simulink model "DualEMDrive3EMRear"  (R2026b)
settings: Solver=VariableStepAuto
undefined symbols (not defined in the file): PlntEMWhlGearRatioRL, PlntEMWhlGearRatioRR
libraries: autolibsharedcoupling x2
settings Model: ModifiedByFormat=The MathWorks, Inc.  Creator=The MathWorks, Inc.  LastModifiedBy=The MathWorks, Inc.
settings OptimizationCC: ReuseModelBlockBuffer=off

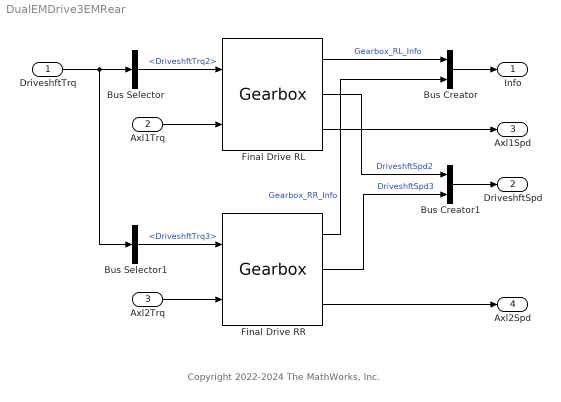
== system DualEMDrive3EMRear ==
  note: Copyright 2022-2024 The MathWorks, Inc.
  DriveshftTrq : Inport
  Axl1Trq : Inport  Port=2
  Axl2Trq : Inport  Port=3
  Bus Creator : BusCreator  Inputs=2
  Bus Creator1 : BusCreator  Inputs=2
  Bus Selector : BusSelector  OutputSignals=DriveshftTrq2
  Bus Selector1 : BusSelector  OutputSignals=DriveshftTrq3
  Final Drive RL : autolibsharedcoupling/Gearbox  port_config=Simulink  input_config=Torque input - velocity output  DiffEffModelPopup=Constant  InterpMethod=Flat  dirSwitch=on  extTamb=off  N=PlntEMWhlGearRatioRL  J1=PlntEMWhlGearInInertiaRL  J2=PlntEMWhlGearOutInertiaRL  b1=PlntEMWhlGearInDampRL  b2=PlntEMWhlGearOutDampRL  theta1_o=0  w1_o=PlntEMWhlGearInInitVelRL  eta=PlntEMWhlGearEffRL  eta_tbl=reshape([0.64 0.76 0.8 0.81 0.83 0.84 0.84 0.56 0.73 0.78 0.8 0.83 0.84 0.84 0.54 0.71 0.77 0.8 0.82 0.84 0.84 0.53 0.71 0.77 0.8 0.83 0.84 0.84 0.51 0.71 0.77 0.8 0.83 0.84 0.85 0.52 0.7 0.77 0.8 0.83 0.84 0.85 0.51 0.71 0.76 0.79 0.83 0.84 0.85 0.5 0.69 0.76 0.79 0.82 0.84 0.85 0.45 0.68 0.75 0.78 0.82 0.84 0.85 0.43 0.67 0.74 0.78 0.81 0.83 0.84 0.38 0.63 0.71 0.75 0.8 0.82 0.83 0.81 0.86 0.88 0.89 0.89 0.89 0.9 0.77 0.85 0.87 0.88 0.89 0.9 0.9 0.72 0.82 0.86 0.87 0.88 0.89 0.9 0.68 0.8 0.84 0.86 0.88 0.89 0.89 0.67 0.8 0.84 0.86 0.88 0.89 0.9 0.67 0.8 0.84 0.86 0.88 0.89 0.9 0.65 0.8 0.84 0.86 0.88 0.89 0.9 0.64 0.79 0.83 0.86 0.88 0.89 0.9 0.63 0.78 0.83 0.86 0.88 0.89 0.9 0.59 0.76 0.82 0.85 0.87 0.89 0.9 0.53 0.73 0.8 0.83 0.86 0.88 0.89], 7, 11, 2)  Trq_bpts=[25, 50, 75, 100, 150, 200, 250]  omega_bpts=[52.4 78.5 105 131 157 183 209 262 314 419 524]  Temp_bpts=[290 358]  Tamb=297.15  blkID=0  aMode=1
      settings: LibrarySourceBlock=autolibcoupling/Gearbox
  Final Drive RR : autolibsharedcoupling/Gearbox  port_config=Simulink  input_config=Torque input - velocity output  DiffEffModelPopup=Constant  InterpMethod=Flat  dirSwitch=on  extTamb=off  N=PlntEMWhlGearRatioRR  J1=PlntEMWhlGearInInertiaRR  J2=PlntEMWhlGearOutInertiaRR  b1=PlntEMWhlGearInDampRR  b2=PlntEMWhlGearOutDampRR  theta1_o=0  w1_o=PlntEMWhlGearInInitVelRR  eta=PlntEMWhlGearEffRR  eta_tbl=reshape([0.64 0.76 0.8 0.81 0.83 0.84 0.84 0.56 0.73 0.78 0.8 0.83 0.84 0.84 0.54 0.71 0.77 0.8 0.82 0.84 0.84 0.53 0.71 0.77 0.8 0.83 0.84 0.84 0.51 0.71 0.77 0.8 0.83 0.84 0.85 0.52 0.7 0.77 0.8 0.83 0.84 0.85 0.51 0.71 0.76 0.79 0.83 0.84 0.85 0.5 0.69 0.76 0.79 0.82 0.84 0.85 0.45 0.68 0.75 0.78 0.82 0.84 0.85 0.43 0.67 0.74 0.78 0.81 0.83 0.84 0.38 0.63 0.71 0.75 0.8 0.82 0.83 0.81 0.86 0.88 0.89 0.89 0.89 0.9 0.77 0.85 0.87 0.88 0.89 0.9 0.9 0.72 0.82 0.86 0.87 0.88 0.89 0.9 0.68 0.8 0.84 0.86 0.88 0.89 0.89 0.67 0.8 0.84 0.86 0.88 0.89 0.9 0.67 0.8 0.84 0.86 0.88 0.89 0.9 0.65 0.8 0.84 0.86 0.88 0.89 0.9 0.64 0.79 0.83 0.86 0.88 0.89 0.9 0.63 0.78 0.83 0.86 0.88 0.89 0.9 0.59 0.76 0.82 0.85 0.87 0.89 0.9 0.53 0.73 0.8 0.83 0.86 0.88 0.89], 7, 11, 2)  Trq_bpts=[25, 50, 75, 100, 150, 200, 250]  omega_bpts=[52.4 78.5 105 131 157 183 209 262 314 419 524]  Temp_bpts=[290 358]  Tamb=297.15  blkID=0  aMode=1
      settings: LibrarySourceBlock=autolibcoupling/Gearbox
  Info : Outport
  DriveshftSpd : Outport  Port=2
  Axl1Spd : Outport  Port=3
  Axl2Spd : Outport  Port=4
  wires:
  Bus Creator/1 -> Info/1
  Axl2Trq/1 -> Final Drive RR/2
  Final Drive RR/3 -> Axl2Spd/1
  Axl1Trq/1 -> Final Drive RL/2
  Final Drive RL/3 -> Axl1Spd/1
  Bus Selector1/1 -> Final Drive RR/1  "<DriveshftTrq3>"
  Final Drive RR/2 -> Bus Creator1/2  "DriveshftSpd3"
  Bus Creator1/1 -> DriveshftSpd/1
  Bus Selector/1 -> Final Drive RL/1  "<DriveshftTrq2>"
  Final Drive RR/1 -> Bus Creator/2  "Gearbox_RR_Info"
  Final Drive RL/2 -> Bus Creator1/1  "DriveshftSpd2"
  Final Drive RL/1 -> Bus Creator/1  "Gearbox_RL_Info"
  DriveshftTrq/1 -> Bus Selector/1, Bus Selector1/1
